simulink subsystem "DebugArray"  (R2025a)
settings: Solver=VariableStepAuto  StartTime=0.0  StopTime=10.0  RelTol=1e-3
undefined symbols (not defined in the file): DiscIntNeverNeededParam
libraries: uavmavlinklib x1
settings Model: Creator=gurt1  LastModifiedBy=17036

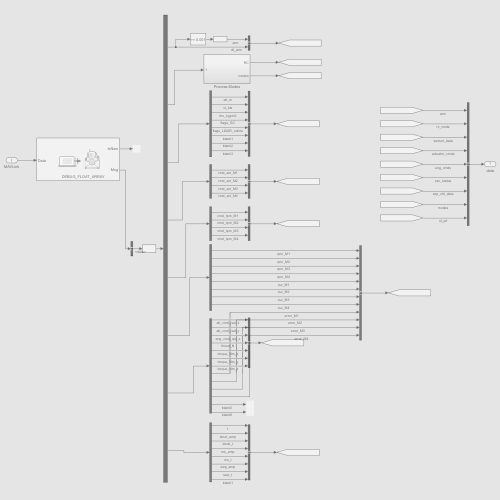
[thumbnail: Simulink's stored preview of the top-level diagram]
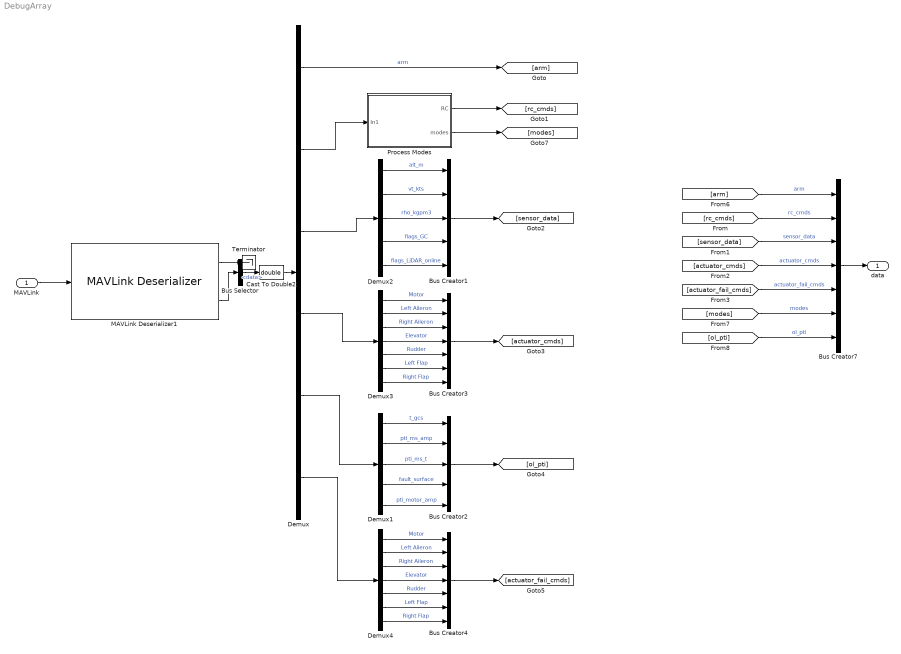
== system DebugArray ==
  MAVLink : Inport
  Bus Creator1 : BusCreator  Inputs=5
  Bus Creator2 : BusCreator  Inputs=5
  Bus Creator3 : BusCreator  Inputs=7
  Bus Creator4 : BusCreator  Inputs=7
  Bus Creator7 : BusCreator  Inputs=7
  Bus Selector : BusSelector  OutputSignals=Payload.data
  Cast To Double2 : DataTypeConversion  OutDataTypeStr=double  SaturateOnIntegerOverflow=off  RndMeth=Floor
  Demux : Demux  Outputs=[1 12 5 7 3 7]
  Demux1 : Demux  Outputs=5
  Demux2 : Demux  Outputs=5
  Demux3 : Demux  Outputs=7
  Demux4 : Demux  Outputs=7
  MAVLink Deserializer1 : uavmavlinklib/MAVLink Deserializer  dialectSource=Select from standard MAVLink dialects  dialect=common.xml  dialectCustom=common.xml  version=2  messageType=DEBUG_FLOAT_ARRAY  inputDataLength=off  SystemIDFilter=off  systemID=1  ComponentIDFilter=off  componentID=1  queueMsg=off  queueMsgSize=50  dropNum=off
  Process Modes : Subsystem
  Terminator : Terminator
  data : Outport
  wires:
  MAVLink/1 -> MAVLink Deserializer1/1
  MAVLink Deserializer1/1 -> Terminator/1
  MAVLink Deserializer1/2 -> Bus Selector/1
  Bus Selector/1 -> Cast To Double2/1  "<data>"
  Demux/3 -> Demux2/1
  Demux/1 -> [arm]  "arm"
  Demux2/1 -> Bus Creator1/1  "alt_m"
  Demux2/2 -> Bus Creator1/2  "vt_kts"
  Demux2/3 -> Bus Creator1/3  "rho_kgpm3"
  Demux2/4 -> Bus Creator1/4  "flags_GC"
  Demux2/5 -> Bus Creator1/5  "flags_LiDAR_online"
  Bus Creator1/1 -> [sensor_data]
  Demux3/4 -> Bus Creator3/4  "Elevator"
  Demux3/3 -> Bus Creator3/3  "Right Aileron"
  Demux3/2 -> Bus Creator3/2  "Left Aileron"
  Demux3/1 -> Bus Creator3/1  "Motor"
  Bus Creator3/1 -> [actuator_cmds]
  Bus Creator7/1 -> data/1
  [rc_cmds] -> Bus Creator7/2  "rc_cmds"
  [sensor_data] -> Bus Creator7/3  "sensor_data"
  [actuator_cmds] -> Bus Creator7/4  "actuator_cmds"
  [actuator_fail_cmds] -> Bus Creator7/5  "actuator_fail_cmds"
  [arm] -> Bus Creator7/1  "arm"
  Demux/2 -> Process Modes/1(In1)
  Process Modes/1(RC) -> [rc_cmds]
  [modes] -> Bus Creator7/6  "modes"
  Process Modes/2(modes) -> [modes]
  Cast To Double2/1 -> Demux/1
  [ol_pti] -> Bus Creator7/7  "ol_pti"
  Demux3/5 -> Bus Creator3/5  "Rudder"
  Demux3/6 -> Bus Creator3/6  "Left Flap"
  Demux3/7 -> Bus Creator3/7  "Right Flap"
  Demux/4 -> Demux3/1
  Demux/5 -> Demux1/1
  Demux1/5 -> Bus Creator2/5  "pti_motor_amp"
  Bus Creator2/1 -> [ol_pti]
  Demux1/1 -> Bus Creator2/1  "t_gcs"
  Demux1/2 -> Bus Creator2/2  "pti_ms_amp"
  Demux1/3 -> Bus Creator2/3  "pti_ms_t"
  Demux1/4 -> Bus Creator2/4  "fault_surface"
  Demux4/7 -> Bus Creator4/7  "Right Flap"
  Demux4/2 -> Bus Creator4/2  "Left Aileron"
  Demux4/1 -> Bus Creator4/1  "Motor"
  Demux4/3 -> Bus Creator4/3  "Right Aileron"
  Bus Creator4/1 -> [actuator_fail_cmds]
  Demux4/5 -> Bus Creator4/5  "Rudder"
  Demux4/4 -> Bus Creator4/4  "Elevator"
  Demux/6 -> Demux4/1
  Demux4/6 -> Bus Creator4/6  "Left Flap"

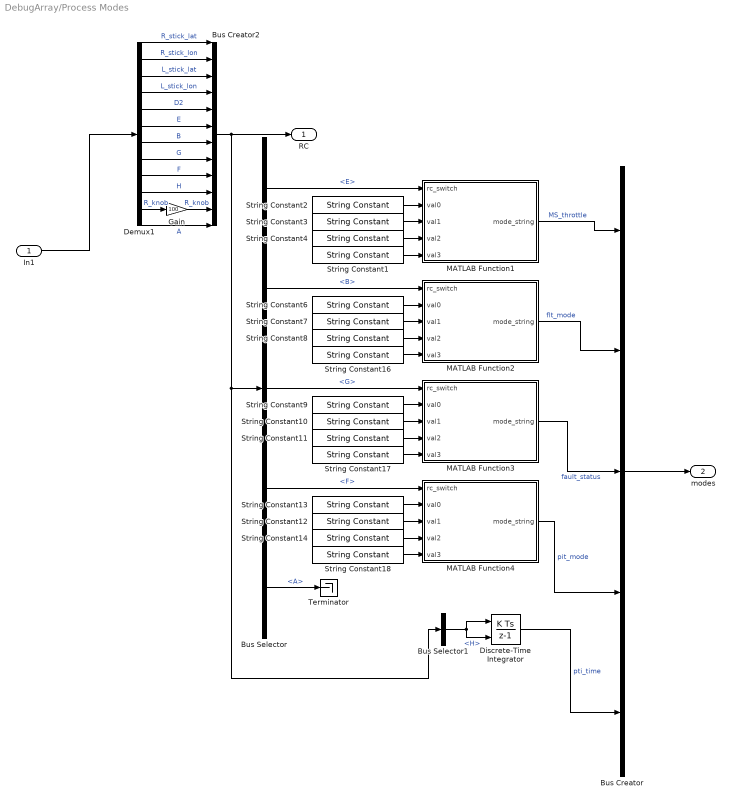
== system DebugArray/Process Modes ==
  In1 : Inport
  Bus Creator : BusCreator  Inputs=5
  Bus Creator2 : BusCreator  Inputs=12
  Bus Selector : BusSelector  OutputSignals=E,B,G,F,A
  Bus Selector1 : BusSelector  OutputSignals=H
  Demux1 : Demux  Outputs=12
  Discrete-Time Integrator : DiscreteIntegrator  ExternalReset=either  SampleTime=-1  ICPrevOutput=DiscIntNeverNeededParam  ICPrevScaledInput=DiscIntNeverNeededParam
  Gain : Gain  Gain=100
  MATLAB Function1 : MATLAB Function  TreatAsAtomicUnit=on
  MATLAB Function2 : MATLAB Function  TreatAsAtomicUnit=on
  MATLAB Function3 : MATLAB Function  TreatAsAtomicUnit=on
  MATLAB Function4 : MATLAB Function  TreatAsAtomicUnit=on
  String Constant{1,16..18} (4 alike) : StringConstant  String="\"Undefined\""
  String Constant10 : StringConstant  String="\"No Fault\""
  String Constant11 : StringConstant  String="\"No Fault\""
  String Constant12 : StringConstant  String="\"FreqSw\""
  String Constant13 : StringConstant  String="\"Doublet\""
  String Constant14 : StringConstant  String="\"Multisin\""
  String Constant2 : StringConstant  String="\"Throttle High\""
  String Constant3 : StringConstant  String="\"Throttle Low\""
  String Constant4 : StringConstant  String="\"Throttle Off\""
  String Constant6 : StringConstant  String="\"Position\""
  String Constant7 : StringConstant  String="\"Altitude\""
  String Constant8 : StringConstant  String="\"Stabilized\""
  String Constant9 : StringConstant  String="\"Fault\""
  Terminator : Terminator
  RC : Outport
  modes : Outport  Port=2
  wires:
  Bus Selector/5 -> Terminator/1  "<A>"
  Demux1/12 -> Bus Creator2/12  "A"
  MATLAB Function1/1(mode_string) -> Bus Creator/1  "MS_throttle"
  String Constant2/1 -> MATLAB Function1/2(val0)
  Bus Selector/1 -> MATLAB Function1/1(rc_switch)  "<E>"
  String Constant4/1 -> MATLAB Function1/4(val2)
  String Constant3/1 -> MATLAB Function1/3(val1)
  String Constant1/1 -> MATLAB Function1/5(val3)
  Discrete-Time Integrator/1 -> Bus Creator/5  "pti_time"
  Bus Selector1/1 -> Discrete-Time Integrator/1, Discrete-Time Integrator/2  "<H>"
  String Constant18/1 -> MATLAB Function4/5(val3)
  String Constant17/1 -> MATLAB Function3/5(val3)
  String Constant16/1 -> MATLAB Function2/5(val3)
  Gain/1 -> Bus Creator2/11  "R_knob"
  String Constant14/1 -> MATLAB Function4/4(val2)
  String Constant12/1 -> MATLAB Function4/3(val1)
  String Constant13/1 -> MATLAB Function4/2(val0)
  String Constant11/1 -> MATLAB Function3/4(val2)
  String Constant10/1 -> MATLAB Function3/3(val1)
  String Constant9/1 -> MATLAB Function3/2(val0)
  String Constant8/1 -> MATLAB Function2/4(val2)
  String Constant7/1 -> MATLAB Function2/3(val1)
  String Constant6/1 -> MATLAB Function2/2(val0)
  MATLAB Function4/1(mode_string) -> Bus Creator/4  "pit_mode"
  MATLAB Function3/1(mode_string) -> Bus Creator/3  "fault_status"
  MATLAB Function2/1(mode_string) -> Bus Creator/2  "flt_mode"
  Bus Creator/1 -> modes/1
  Bus Selector/4 -> MATLAB Function4/1(rc_switch)  "<F>"
  Bus Selector/3 -> MATLAB Function3/1(rc_switch)  "<G>"
  Bus Selector/2 -> MATLAB Function2/1(rc_switch)  "<B>"
  Bus Creator2/1 -> RC/1, Bus Selector/1, Bus Selector1/1
  In1/1 -> Demux1/1
  Demux1/6 -> Bus Creator2/6  "E"
  Demux1/1 -> Bus Creator2/1  "R_stick_lat"
  Demux1/5 -> Bus Creator2/5  "D2"
  Demux1/9 -> Bus Creator2/9  "F"
  Demux1/3 -> Bus Creator2/3  "L_stick_lat"
  Demux1/11 -> Gain/1  "R_knob"
  Demux1/7 -> Bus Creator2/7  "B"
  Demux1/8 -> Bus Creator2/8  "G"
  Demux1/4 -> Bus Creator2/4  "L_stick_lon"
  Demux1/2 -> Bus Creator2/2  "R_stick_lon"
  Demux1/10 -> Bus Creator2/10  "H"

== matlab function DebugArray/Process Modes/MATLAB Function1 ==
  data: rc_switch input; mode_string output; val0 input; val1 input; val2 input; val3 input
function mode_string = process_mode(rc_switch, val0, val1, val2, val3)

mode_string = process_mode(rc_switch, val0, val1, val2,val3);

== matlab function DebugArray/Process Modes/MATLAB Function2 ==
  data: rc_switch input; mode_string output; val0 input; val1 input; val2 input; val3 input
function mode_string = process_mode(rc_switch, val0, val1, val2, val3)

mode_string = process_mode(rc_switch, val0, val1, val2,val3);

== matlab function DebugArray/Process Modes/MATLAB Function3 ==
  data: rc_switch input; mode_string output; val0 input; val1 input; val2 input; val3 input
function mode_string = process_mode(rc_switch, val0, val1, val2, val3)

mode_string = process_mode(rc_switch, val0, val1, val2,val3);

== matlab function DebugArray/Process Modes/MATLAB Function4 ==
  data: rc_switch input; mode_string output; val0 input; val1 input; val2 input; val3 input
function mode_string = process_mode(rc_switch, val0, val1, val2, val3)

mode_string = process_mode(rc_switch, val0, val1, val2,val3);
